simulink model "DueSerbatoiEasy"  (R2022b)
settings: Solver=VariableStepAuto  StartTime=0.0  StopTime=150  RelTol=1e-3
values from neighbouring files (symbols this model uses):
  C1 = 1    [DueSerbatoiEasy_values.m]    (also in DueSerbatoiSS.m)
  C2 = 1    [DueSerbatoiEasy_values.m]    (also in DueSerbatoiSS.m)
  L = 1    [DueSerbatoiEasy_values.m]    (also in DueSerbatoiSS.m)
  Q1 = 1    [DueSerbatoiSS.m]
  R = 1    [DueSerbatoiEasy_values.m]    (also in DueSerbatoiSS.m)
settings Model: Creator=giuli  LastModifiedBy=giuli

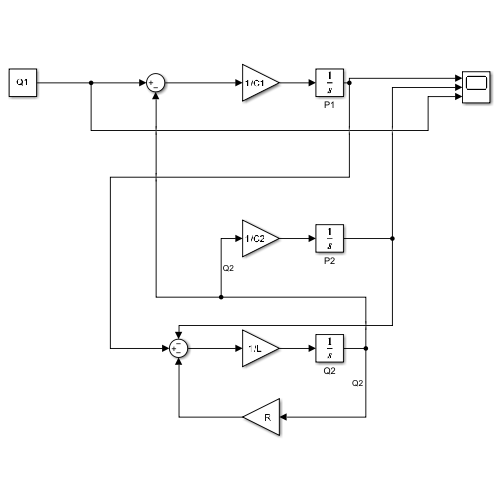
[thumbnail: Simulink's stored preview of the top-level diagram]
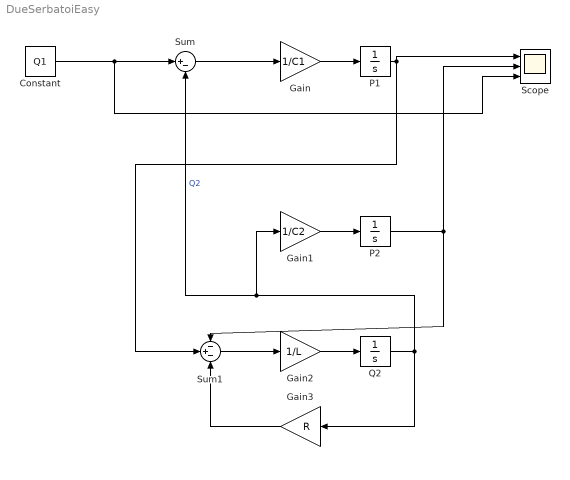
== system DueSerbatoiEasy ==
  Constant : Constant  Value=Q1
  Gain : Gain  Gain=1/C1
  Gain1 : Gain  Gain=1/C2
  Gain2 : Gain  Gain=1/L
  Gain3 : Gain  Gain=R
  P1 : Integrator
  P2 : Integrator
  Q2 : Integrator
  Scope : Scope  NumInputPorts=3
  Sum : Sum  Inputs=|+-
  Sum1 : Sum  Inputs=-+-
  wires:
  Gain/1 -> P1/1
  Sum/1 -> Gain/1
  Constant/1 -> Scope/3, Sum/1
  Gain1/1 -> P2/1
  Gain2/1 -> Q2/1
  Q2/1 -> Gain3/1, Gain1/1, Sum/2  "Q2"
  Sum1/1 -> Gain2/1
  P2/1 -> Sum1/1, Scope/2
  P1/1 -> Sum1/2, Scope/1
  Gain3/1 -> Sum1/3
